simulink model "PID_ASR_PID_ACR"  (R2020a)
settings: Solver=ode45  StartTime=0.0  StopTime=10.0  MaxStep=1e-5  RelTol=1e-3
settings Model: Creator=78253  LastModifiedBy=78253

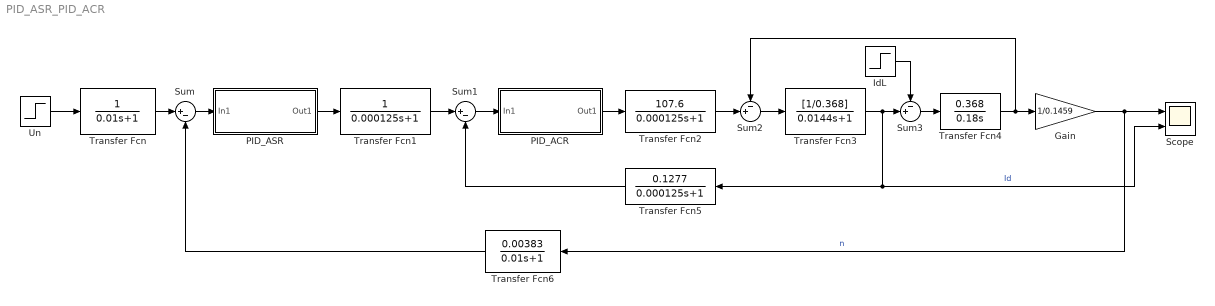
== system PID_ASR_PID_ACR ==
  Gain : Gain  Gain=1/0.1459
  IdL : Step  Time=0  After=52.2  SampleTime=0
  PID_ACR : Subsystem
  PID_ASR : Subsystem
  Scope : Scope  NumInputPorts=2
  Sum : Sum  Inputs=|+-
  Sum1 : Sum  Inputs=|+-
  Sum2 : Sum  Inputs=-+|
  Sum3 : Sum  Inputs=-+|
  Transfer Fcn : TransferFcn  Denominator=[0.01 1]
  Transfer Fcn1 : TransferFcn  Denominator=[0.000125 1]
  Transfer Fcn2 : TransferFcn  Numerator=[107.6]  Denominator=[0.000125 1]
  Transfer Fcn3 : TransferFcn  Numerator=[1/0.368]  Denominator=[0.0144 1]
  Transfer Fcn4 : TransferFcn  Numerator=[0.368]  Denominator=[0.18 0]
  Transfer Fcn5 : TransferFcn  Numerator=[0.1277]  Denominator=[0.000125 1]
  Transfer Fcn6 : TransferFcn  Numerator=[0.00383]  Denominator=[0.01 1]
  Un : Step  Time=0  After=10  SampleTime=0
  wires:
  Un/1 -> Transfer Fcn/1
  Transfer Fcn/1 -> Sum/1
  Sum/1 -> PID_ASR/1(In1)
  PID_ASR/1(Out1) -> Transfer Fcn1/1
  Transfer Fcn1/1 -> Sum1/1
  Sum1/1 -> PID_ACR/1(In1)
  PID_ACR/1(Out1) -> Transfer Fcn2/1
  Transfer Fcn2/1 -> Sum2/2
  Sum2/1 -> Transfer Fcn3/1
  Transfer Fcn3/1 -> Transfer Fcn5/1, Scope/2, Sum3/2  "Id"
  IdL/1 -> Sum3/1
  Sum3/1 -> Transfer Fcn4/1
  Transfer Fcn4/1 -> Sum2/1, Gain/1
  Gain/1 -> Transfer Fcn6/1, Scope/1  "n"
  Transfer Fcn6/1 -> Sum/2
  Transfer Fcn5/1 -> Sum1/2

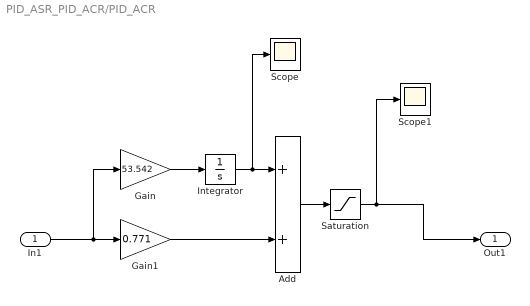
== system PID_ASR_PID_ACR/PID_ACR ==
  In1 : Inport
  Add : Sum
  Gain : Gain  Gain=53.542
  Gain1 : Gain  Gain=0.771
  Integrator : Integrator  LimitOutput=on  UpperSaturationLimit=5  LowerSaturationLimit=-5
  Saturation : Saturate  UpperLimit=5  LowerLimit=-5
  Scope : Scope
  Scope1 : Scope
  Out1 : Outport
  wires:
  In1/1 -> Gain/1, Gain1/1
  Gain1/1 -> Add/2
  Add/1 -> Saturation/1
  Gain/1 -> Integrator/1
  Saturation/1 -> Out1/1, Scope1/1
  Integrator/1 -> Scope/1, Add/1

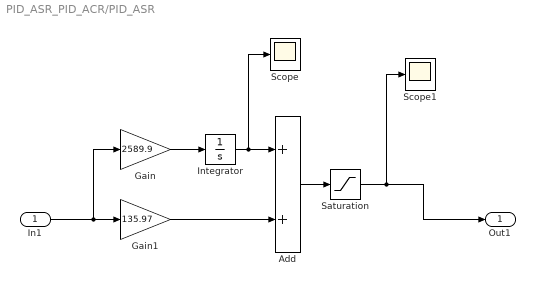
== system PID_ASR_PID_ACR/PID_ASR ==
  In1 : Inport
  Add : Sum
  Gain : Gain  Gain=2589.9
  Gain1 : Gain  Gain=135.97
  Integrator : Integrator  LimitOutput=on  UpperSaturationLimit=10  LowerSaturationLimit=-10
  Saturation : Saturate  UpperLimit=10  LowerLimit=-10
  Scope : Scope
  Scope1 : Scope
  Out1 : Outport
  wires:
  In1/1 -> Gain/1, Gain1/1
  Gain/1 -> Integrator/1
  Gain1/1 -> Add/2
  Integrator/1 -> Scope/1, Add/1
  Add/1 -> Saturation/1
  Saturation/1 -> Scope1/1, Out1/1
